simulink model "IO601queueloopback"  (R2012a)
settings: Solver=FixedStepDiscrete  SolverMode=SingleTasking  StartTime=0.0  StopTime=inf  RelTol=1e-3
libraries: canmsglib x4, speedgoatlib_IO601 x4, xpclib x2, simulink x1
Description:
  | 7.14.0.739 (R2012a)
settings Model: BufferReuse=off  Creator=dkuratli  LastModifiedBy=lab3
settings SolverCC: EnableConcurrentExecution=on
settings DataIOCC: LimitDataPoints=on  SaveFormat=Array  SignalLoggingSaveFormat=ModelDataLogs  ReturnWorkspaceOutputs=off
settings OptimizationCC: BlockReduction=off  OptimizeBlockIOStorage=off  BufferReuse=off  ExpressionFolding=off  ExpressionDepthLimit=2147483647  LocalBlockOutputs=off  LifeSpan=inf  SimCompilerOptimization=Off
settings DebuggingCC: UnderspecifiedInitializationDetection=Classic  MergeDetectMultiDrivingBlocksExec=none  SolverPrmCheckMsg=warning  FcnCallInpInsideContextMsg=Use local settings  FrameProcessingCompatibilityMsg=warning  StateNameClashWarn=warning  SFUnexpectedBacktrackingDiag=warning  SFNoUnconditionalDefaultTransitionDiag=warning
settings HardwareCC: ProdBitPerPointer=32  ProdLargestAtomicFloat=None  ProdWordSize=32  ProdHWDeviceType=Generic->32-bit x86 compatible
settings ModelReferenceCC: PropagateSignalLabelsOutOfModel=off
settings SFSimCC: SimUseLocalCustomCode=off
settings RTWCC: SystemTargetFile=xpctarget.tlc  TemplateMakefile=xpc_default_tmf  Description=Simulink Real-Time  RTWVerbose=off  ProcessScript=xpctarget_make_rtw_hook  RTWUseLocalCustomCode=off  RTWCompilerOptimization=On
settings xpcTargetCC: TargetFcnLib=ansi_tfl_table_tmw.mat  CodeReplacementLibrary=XPC_BLAS  ParMdlRefBuildCompliant=on  ConcurrentExecutionCompliant=on  CombineSignalStateStructs=off  GRTInterface=on  GenerateAllocFcn=off  xPCTaskExecutionProfile=off  xPCRL32EventNumber=5000  xPCLoadParamSetFile=off  xPCConcurrentTasks=off  xPCEnableSFAnimation=off

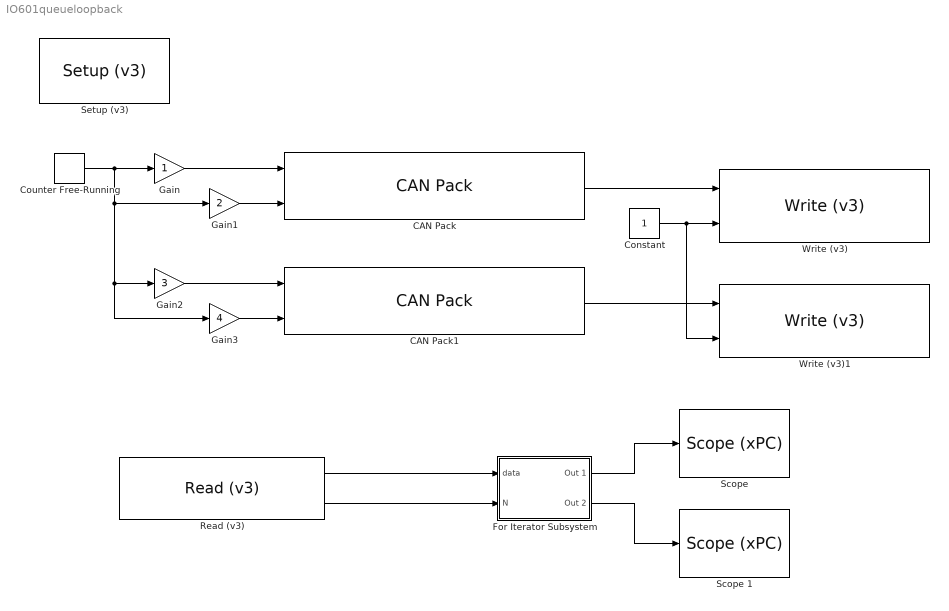
== system IO601queueloopback ==
  CAN Pack : canmsglib/CAN Pack  MsgList=(none)  MsgName=Message20  MsgIDType=Standard (11-bit identifier)  MsgIdentifier=32  MsgLength=4  SignalInfo=Signal1$0$16$1$1$1$0$1$0$-Inf$Inf$#Signal2$16$16$1$1$1$0$1$0$-Inf$Inf$#  NSignals=2  StartBits=str2num('[int32(0);int32(16)]')  SignalSizes=str2num('[int32(16);int32(16)]')  ByteOrders=str2num('[int32(1);int32(1)]')  DataTypes=str2num('[int32(1);int32(1)]')  MultiplexTypes=str2num('[int32(1);int32(1)]')  MultiplexValues=str2num('[double(0);double(0)]')  Factors=str2num('[double(1);double(1)]')  Offsets=str2num('[double(0);double(0)]')  Minimums=str2num('[double(-Inf);double(-Inf)]')  Maximums=str2num('[double(Inf);double(Inf)]')  Remote=off
      settings: DataFormat=manually specified signals
  CAN Pack1 : canmsglib/CAN Pack  MsgList=(none)  MsgName=Message21  MsgIDType=Standard (11-bit identifier)  MsgIdentifier=33  MsgLength=4  SignalInfo=Signal3$0$16$1$1$1$0$1$0$-Inf$Inf$#Signal4$16$16$1$1$1$0$1$0$-Inf$Inf$#  NSignals=2  StartBits=str2num('[int32(0);int32(16)]')  SignalSizes=str2num('[int32(16);int32(16)]')  ByteOrders=str2num('[int32(1);int32(1)]')  DataTypes=str2num('[int32(1);int32(1)]')  MultiplexTypes=str2num('[int32(1);int32(1)]')  MultiplexValues=str2num('[double(0);double(0)]')  Factors=str2num('[double(1);double(1)]')  Offsets=str2num('[double(0);double(0)]')  Minimums=str2num('[double(-Inf);double(-Inf)]')  Maximums=str2num('[double(Inf);double(Inf)]')  Remote=off
      settings: DataFormat=manually specified signals
  Constant : Constant
  Counter Free-Running : simulink/Sources/Counter Free-Running  NumBits=16  tsamp=0.001
  For Iterator Subsystem : Subsystem  TreatAsAtomicUnit=on
  Gain : Gain  OutDataTypeStr=Inherit: Inherit via back propagation
  Gain1 : Gain  Gain=2  OutDataTypeStr=Inherit: Inherit via back propagation
  Gain2 : Gain  Gain=3  OutDataTypeStr=Inherit: Inherit via back propagation
  Gain3 : Gain  Gain=4  OutDataTypeStr=Inherit: Inherit via back propagation
  Read (v3) : speedgoatlib_IO601/Read (v3)  id=1  outputFormat=Vector of CAN_MESSAGE  port1=on  port2=off  depth1=4  depth2=4  sampletime=0.001  pciSlot=-1
  "Scope " : xpclib/Misc./Scope (xPC)   scopeno=1  scopetype=Target  autostart=on  viewmode=Numerical  formatstr='%15.6f'  grid=on  ylimits=[0,0]  nosamples=3  noprepostsamples=0  interleave=1  triggermode=FreeRun  triggersignal=1  trigsignalfromport=off  triggerlevel=0.0  triggerslope=Either  triggerscope=1  triggersample=0  filename=data.dat  mode=Lazy  writesize=512  autorestart=off  dynamicfilemode=off  maxwritefilesize=512*1024^2
  Scope 1 : xpclib/Misc./Scope (xPC)   scopeno=2  scopetype=Target  autostart=on  viewmode=Numerical  formatstr='%15.6f'  grid=on  ylimits=[0,0]  nosamples=3  noprepostsamples=0  interleave=1  triggermode=FreeRun  triggersignal=1  trigsignalfromport=off  triggerlevel=0.0  triggerslope=Either  triggerscope=1  triggersample=0  filename=data.dat  mode=Lazy  writesize=512  autorestart=off  dynamicfilemode=off  maxwritefilesize=512*1024^2
  Setup (v3) : speedgoatlib_IO601/Setup (v3)  id=1  can1enable=on  can1bus=Highspeed  can1Baudrate=1 MBaud  can1UserBR=[1,1,5,2]  stdAcc1=[0,0,0,0]  extAcc1=[0,0,0,0]  can2enable=on  can2bus=Highspeed  can2Baudrate=1 MBaud  can2UserBR=[1,1,5,2]  stdAcc2=[0,0,0,0]  extAcc2=[0,0,0,0]  pciSlot=-1
  Write (v3) : speedgoatlib_IO601/Write (v3)  Priority=1  id=1  sampletime=0.002  pciSlot=-1  inputType=CAN_MESSAGE plus count  port=2  maxMsg=1  status=off  init=[]  term=[]
  Write (v3)1 : speedgoatlib_IO601/Write (v3)  Priority=1  id=1  sampletime=0.001  pciSlot=-1  inputType=CAN_MESSAGE plus count  port=2  maxMsg=1  status=off  init=[]  term=[]
  wires:
  Counter Free-Running/1 -> Gain3/1, Gain2/1, Gain1/1, Gain/1
  CAN Pack/1 -> Write (v3)/1
  CAN Pack1/1 -> Write (v3)1/1
  Gain/1 -> CAN Pack/1
  Gain1/1 -> CAN Pack/2
  Gain2/1 -> CAN Pack1/1
  Gain3/1 -> CAN Pack1/2
  Constant/1 -> Write (v3)1/2, Write (v3)/2
  Read (v3)/1 -> For Iterator Subsystem/1(data)
  Read (v3)/2 -> For Iterator Subsystem/2(N)
  For Iterator Subsystem/1(Out 1) -> "Scope "/1
  For Iterator Subsystem/2(Out 2) -> Scope 1/1

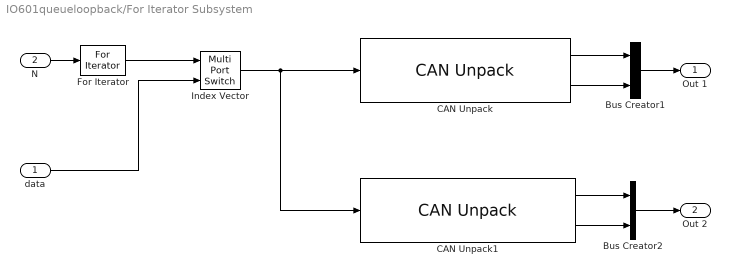
== system IO601queueloopback/For Iterator Subsystem ==
  data : Inport
  N : Inport  Port=2
  Bus Creator1 : BusCreator  Inputs=2
  Bus Creator2 : BusCreator  Inputs=2
  CAN Unpack : canmsglib/CAN Unpack  MsgList=(none)  MsgName=Message20  MsgIDType=Standard (11-bit identifier)  MsgIdentifier=32  MsgLength=4  SignalInfo=Signal1$0$16$1$1$1$0$1$0$-Inf$Inf$#Signal2$16$16$1$1$1$0$1$0$-Inf$Inf$#  NSignals=2  IDPort=off  TimestampPort=off  ErrorPort=off  RemotePort=off  LengthPort=off  StatusPort=off  StartBits=str2num('[int32(0);int32(16)]')  SignalSizes=str2num('[int32(16);int32(16)]')  ByteOrders=str2num('[int32(1);int32(1)]')  DataTypes=str2num('[int32(1);int32(1)]')  MultiplexTypes=str2num('[int32(1);int32(1)]')  MultiplexValues=str2num('[double(0);double(0)]')  Factors=str2num('[double(1);double(1)]')  Offsets=str2num('[double(0);double(0)]')  Minimums=str2num('[double(-Inf);double(-Inf)]')  Maximums=str2num('[double(Inf);double(Inf)]')
  CAN Unpack1 : canmsglib/CAN Unpack  MsgList=(none)  MsgName=Message21  MsgIDType=Standard (11-bit identifier)  MsgIdentifier=33  MsgLength=4  SignalInfo=Signal3$0$16$1$1$1$0$1$0$-Inf$Inf$#Signal4$16$16$1$1$1$0$1$0$-Inf$Inf$#  NSignals=2  IDPort=off  TimestampPort=off  ErrorPort=off  RemotePort=off  LengthPort=off  StatusPort=off  StartBits=str2num('[int32(0);int32(16)]')  SignalSizes=str2num('[int32(16);int32(16)]')  ByteOrders=str2num('[int32(1);int32(1)]')  DataTypes=str2num('[int32(1);int32(1)]')  MultiplexTypes=str2num('[int32(1);int32(1)]')  MultiplexValues=str2num('[double(0);double(0)]')  Factors=str2num('[double(1);double(1)]')  Offsets=str2num('[double(0);double(0)]')  Minimums=str2num('[double(-Inf);double(-Inf)]')  Maximums=str2num('[double(Inf);double(Inf)]')
  For Iterator : ForIterator  IterationSource=external  IterationLimit=20  IterationVariableDataType=int8
  Index Vector : MultiPortSwitch  Inputs=1
  Out 1 : Outport
  Out 2 : Outport  Port=2
  wires:
  Index Vector/1 -> CAN Unpack1/1, CAN Unpack/1
  Bus Creator1/1 -> Out 1/1
  For Iterator/1 -> Index Vector/1
  data/1 -> Index Vector/2
  Bus Creator2/1 -> Out 2/1
  CAN Unpack/1 -> Bus Creator1/1
  CAN Unpack/2 -> Bus Creator1/2
  CAN Unpack1/1 -> Bus Creator2/1
  CAN Unpack1/2 -> Bus Creator2/2
  N/1 -> For Iterator/1
